simulink model "codeGen"  (R2025b)
settings: configuration reference "code" (kept outside this file)
settings Model: DataDictionary=test.sldd  Creator=rpumpo  LastModifiedBy=rpumpo
settings ConfigSetRef: SourceName=code

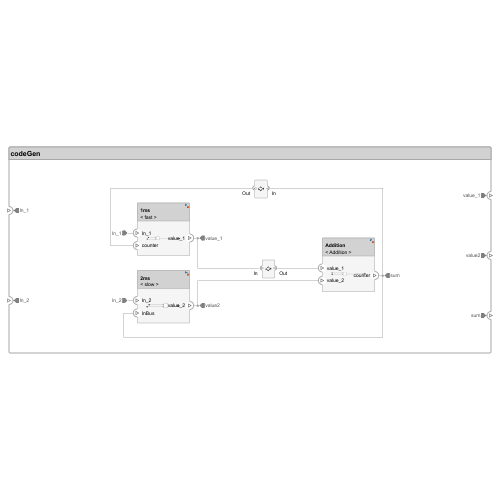
[thumbnail: Simulink's stored preview of the top-level diagram]
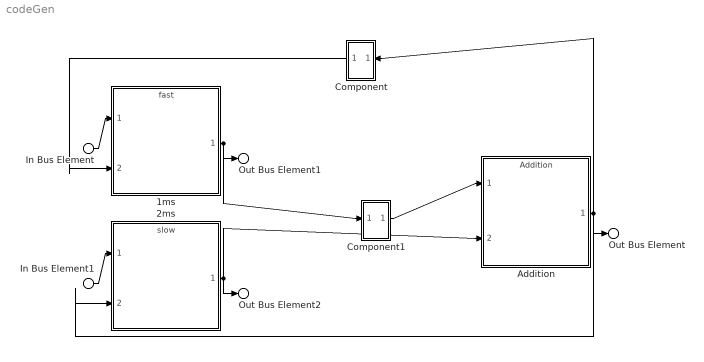
== system codeGen ==
  In Bus Element : Inport  PortName=In_1
  In Bus Element1 : Inport  Port=2  PortName=In_2
  1ms : ModelReference  ModelNameDialog=fast  ModelReferenceVersion=1.8
      settings: PortSchema="{\"entries\":[{\"content\":{\"headerSize\":38,\"margin\":15,\"minimumSpacing\":25,\"sides\":[{\"content\":{\"connectorIds\":[\"In1\",\"In2\"]},\"type\":\"ConnectorPlacement.EquallySpacedRectSide\",\"uuid\":\"d2c06549-0a8a-4f10-824f-4b564c223fac\"},{\"content\":{\"connectorIds\":[\"Out1\"],\"side\":\"RIGHT\"},\"type\":\"ConnectorPlacement.EquallySpacedRectSide\",\"uuid\":\"7f3d62f4-d07f-47a7-8f95-415a6e5f3cea\"},{\"content\":{\"side\":\"TOP\"},\"type\":\"ConnectorPlacement.EquallySpacedRectSide\",\"uuid\":\"2a783486-aeab-4ab5-a645-d34808ec0d54\"}]},\"type\":\"ConnectorPlacement.EquallySpacedConnector\",\"uuid\":\"7a5c9441-6c99-4aab-b214-58c8e6885b4c\"}],\"packageUris\":[\"http://schema.mathworks.com/mf0/Connector/R2020b\"],\"version\":\"1.0\"}"
  2ms : ModelReference  ModelNameDialog=slow  SimulationMode=Normal  ModelReferenceVersion=1.9
      settings: PortSchema="{\"entries\":[{\"content\":{\"headerSize\":38,\"margin\":15,\"minimumSpacing\":25,\"sides\":[{\"content\":{\"connectorIds\":[\"In1\",\"In2\"]},\"type\":\"ConnectorPlacement.EquallySpacedRectSide\",\"uuid\":\"d2c06549-0a8a-4f10-824f-4b564c223fac\"},{\"content\":{\"connectorIds\":[\"Out1\"],\"side\":\"RIGHT\"},\"type\":\"ConnectorPlacement.EquallySpacedRectSide\",\"uuid\":\"7f3d62f4-d07f-47a7-8f95-415a6e5f3cea\"},{\"content\":{\"side\":\"TOP\"},\"type\":\"ConnectorPlacement.EquallySpacedRectSide\",\"uuid\":\"2a783486-aeab-4ab5-a645-d34808ec0d54\"}]},\"type\":\"ConnectorPlacement.EquallySpacedConnector\",\"uuid\":\"7a5c9441-6c99-4aab-b214-58c8e6885b4c\"}],\"packageUris\":[\"http://schema.mathworks.com/mf0/Connector/R2020b\"],\"version\":\"1.0\"}"
  Addition : ModelReference  ModelNameDialog=Addition  SimulationMode=Normal  ModelReferenceVersion=1.6
      settings: PortSchema="{\"entries\":[{\"content\":{\"headerSize\":38,\"margin\":15,\"minimumSpacing\":25,\"sides\":[{\"content\":{\"connectorIds\":[\"In1\",\"In2\"]},\"type\":\"ConnectorPlacement.EquallySpacedRectSide\",\"uuid\":\"d2c06549-0a8a-4f10-824f-4b564c223fac\"},{\"content\":{\"connectorIds\":[\"Out1\"],\"side\":\"RIGHT\"},\"type\":\"ConnectorPlacement.EquallySpacedRectSide\",\"uuid\":\"7f3d62f4-d07f-47a7-8f95-415a6e5f3cea\"},{\"content\":{\"side\":\"TOP\"},\"type\":\"ConnectorPlacement.EquallySpacedRectSide\",\"uuid\":\"2a783486-aeab-4ab5-a645-d34808ec0d54\"}]},\"type\":\"ConnectorPlacement.EquallySpacedConnector\",\"uuid\":\"7a5c9441-6c99-4aab-b214-58c8e6885b4c\"}],\"packageUris\":[\"http://schema.mathworks.com/mf0/Connector/R2020b\"],\"version\":\"1.0\"}"
  Component : Subsystem
      settings: PortSchema="{\"entries\":[{\"content\":{\"margin\":10,\"minimumSpacing\":15,\"sides\":[{\"content\":{\"connectorIds\":[\"Out1\"]},\"type\":\"ConnectorPlacement.EquallySpacedRectSide\",\"uuid\":\"863a0b16-e36b-44d6-9477-1468a80c696d\"},{\"content\":{\"connectorIds\":[\"In1\"],\"side\":\"RIGHT\"},\"type\":\"ConnectorPlacement.EquallySpacedRectSide\",\"uuid\":\"ac9067ee-3fe6-46b1-b4d3-b466d54413ae\"},{\"content\":{\"side\":\"TOP\"},\"type\":\"ConnectorPlacement.EquallySpacedRectSide\",\"uuid\":\"d4aa2d7a-4362-47d2-9788-fc41168b683c\"}]},\"type\":\"ConnectorPlacement.EquallySpacedConnector\",\"uuid\":\"884a1123-87f2-4a92-8ca9-5d4169531818\"}],\"packageUris\":[\"http://schema.mathworks.com/mf0/Connector/R2020b\"],\"version\":\"1.0\"}"
  Component1 : Subsystem
      settings: PortSchema="{\"entries\":[{\"content\":{\"margin\":10,\"minimumSpacing\":15,\"sides\":[{\"content\":{\"connectorIds\":[\"In1\"]},\"type\":\"ConnectorPlacement.EquallySpacedRectSide\",\"uuid\":\"863a0b16-e36b-44d6-9477-1468a80c696d\"},{\"content\":{\"connectorIds\":[\"Out1\"],\"side\":\"RIGHT\"},\"type\":\"ConnectorPlacement.EquallySpacedRectSide\",\"uuid\":\"ac9067ee-3fe6-46b1-b4d3-b466d54413ae\"},{\"content\":{\"side\":\"TOP\"},\"type\":\"ConnectorPlacement.EquallySpacedRectSide\",\"uuid\":\"d4aa2d7a-4362-47d2-9788-fc41168b683c\"}]},\"type\":\"ConnectorPlacement.EquallySpacedConnector\",\"uuid\":\"884a1123-87f2-4a92-8ca9-5d4169531818\"}],\"packageUris\":[\"http://schema.mathworks.com/mf0/Connector/R2020b\"],\"version\":\"1.0\"}"
  Out Bus Element1 : Outport  PortName=value_1
  Out Bus Element2 : Outport  Port=2  PortName=value2
  Out Bus Element : Outport  Port=3  PortName=sum
  wires:
  In Bus Element/1 -> 1ms/1
  In Bus Element1/1 -> 2ms/1
  Addition/1 -> 2ms/2, Out Bus Element/1, Component/1(In)
  2ms/1 -> Addition/2, Out Bus Element2/1
  1ms/1 -> Out Bus Element1/1, Component1/1(In)
  Component/1(Out) -> 1ms/2
  Component1/1(Out) -> Addition/1

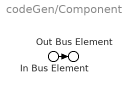
== system codeGen/Component ==
  In Bus Element : Inport  PortName=In
  Out Bus Element : Outport  PortName=Out
  wires:
  In Bus Element/1 -> Out Bus Element/1

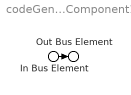
== system codeGen/Component1 ==
  In Bus Element : Inport  PortName=In
  Out Bus Element : Outport  PortName=Out
  wires:
  In Bus Element/1 -> Out Bus Element/1
